simulink library "realFlowEnvironment_cl"  (R2018b)
settings: Solver=VariableStepAuto  StartTime=0.0  StopTime=10.0  RelTol=1e-3
settings Model: Creator=mcobb  LastModifiedBy=mcobb

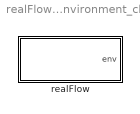
== system realFlowEnvironment_cl ==
  realFlow : Subsystem

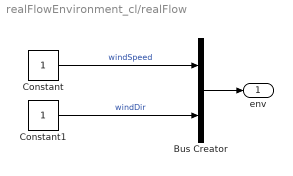
== system realFlowEnvironment_cl/realFlow ==
  Bus Creator : BusCreator  Inputs=2
  Constant : Constant
  Constant1 : Constant
  env : Outport  OutDataTypeStr=Bus: envBus
  wires:
  Bus Creator/1 -> env/1
  Constant/1 -> Bus Creator/1  "windSpeed"
  Constant1/1 -> Bus Creator/2  "windDir"
